simulink model "simulation_control_LQR_azioneintegrale_WP2"  (R2023b)
settings: Solver=VariableStepAuto  StartTime=0.0  StopTime=100  RelTol=1e-3
values from neighbouring files (symbols this model uses):
  K = [k1 k2 ki]    [WP2.m]
settings Model: Creator=giova  LastModifiedBy=giova

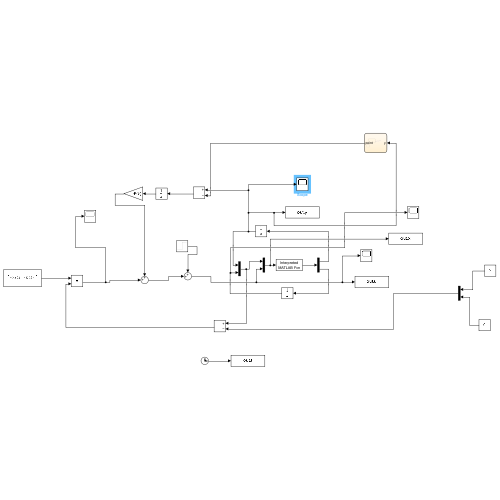
[thumbnail: Simulink's stored preview of the top-level diagram]
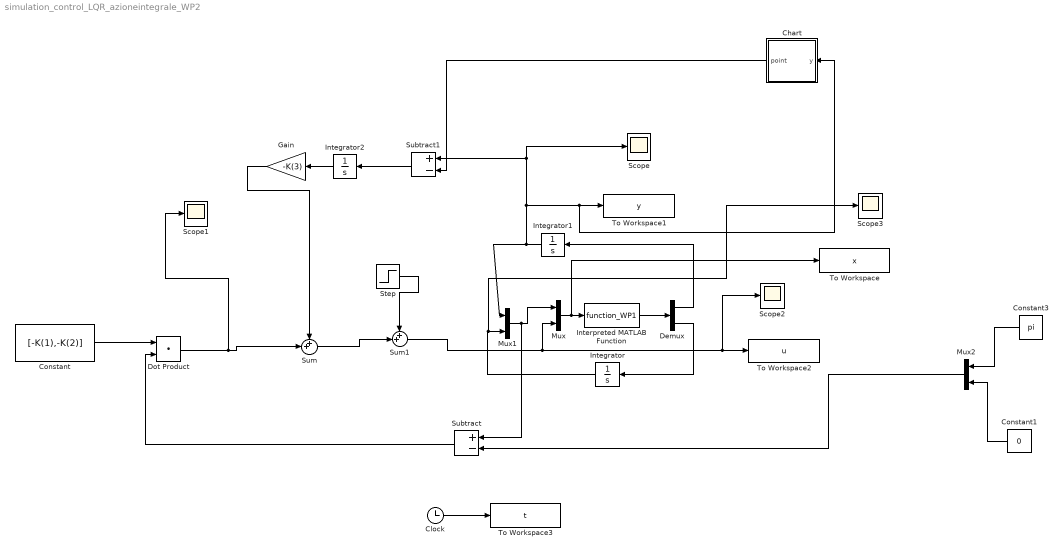
== system simulation_control_LQR_azioneintegrale_WP2 ==
  Chart : Stateflow chart  TreatAsAtomicUnit=on
  Clock : Clock
  Constant : Constant  Value=[-K(1),-K(2)]
  Constant1 : Constant  Value=0
  Constant3 : Constant  Value=pi
  Demux : Demux  Outputs=2
  Dot Product : DotProduct  OutDataTypeStr=Inherit: Inherit via internal rule
  Gain : Gain  Gain=-K(3)
  Integrator : Integrator
  Integrator1 : Integrator
  Integrator2 : Integrator
  Interpreted MATLAB Function : MATLABFcn  MATLABFcn=function_WP1  OutputDimensions=2
  Mux : Mux  Inputs=2
  Mux1 : Mux  Inputs=2
  Mux2 : Mux  Inputs=2
  Scope{,1..3} (4 alike) : Scope
  Step : Step  Time=5  After=+1000  SampleTime=0
  Subtract : Sum  Inputs=+-
  Subtract1 : Sum  Inputs=+-
  Sum : Sum  Inputs=++|
  Sum1 : Sum  Inputs=++|
  To Workspace : ToWorkspace  VariableName=x  SampleTime=-1
  To Workspace1 : ToWorkspace  VariableName=y  SampleTime=-1
  To Workspace2 : ToWorkspace  VariableName=u  SampleTime=-1
  To Workspace3 : ToWorkspace  VariableName=t  SampleTime=-1
  wires:
  Dot Product/1 -> Sum/2, Scope1/1
  Constant/1 -> Dot Product/1
  Integrator/1 -> Scope3/1, Mux1/2
  Demux/2 -> Integrator/1
  Mux1/1 -> Subtract/1, Mux/1
  Clock/1 -> To Workspace3/1
  Subtract/1 -> Dot Product/2
  Integrator1/1 -> Subtract1/1, Scope/1, Chart/1(y), To Workspace1/1, Mux1/1
  Demux/1 -> Integrator1/1
  Mux/1 -> To Workspace/1, Interpreted MATLAB Function/1
  Interpreted MATLAB Function/1 -> Demux/1
  Sum/1 -> Sum1/2
  Sum1/1 -> Mux/2, Scope2/1, To Workspace2/1
  Subtract1/1 -> Integrator2/1
  Integrator2/1 -> Gain/1
  Chart/1(point) -> Subtract1/2
  Gain/1 -> Sum/1
  Step/1 -> Sum1/1
  Constant1/1 -> Mux2/2
  Mux2/1 -> Subtract/2
  Constant3/1 -> Mux2/1

== stateflow chart simulation_control_LQR_azioneintegrale_WP2/Chart ==
  state Normal_situation
    en:
    point=fix(y/(pi))*pi+pi*sign(y)
    a=(point/pi)+1
    b=(point/pi)-1
  state initial
    en:
    a=2
    b=0
  Normal_situation -> Normal_situation : [(y>=a*pi || y<=b*pi)]
  initial -> Normal_situation
  (default) -> initial
  data: point output; a local; b local; y input
